simulink subsystem "ModeloSistemaNL"  (R2026a)
settings: Solver=VariableStepAuto
values from neighbouring files (symbols this model uses):
  alpha_Cu = 3.9e-3    (= 0.0039)    [coeficientes.m]
  b_eq = b_m + b_l/(r_m2l^2)    (= 2.19444444444e-05)    [coeficientes.m]
  C_ts = 0.818    [coeficientes.m]
  g = 9.80665    [coeficientes.m]
  J_eq = J_m + J_l/(r_m2l^2)    (= 4.58263888889e-05)    [coeficientes.m]
  k_l = 0.1    [coeficientes.m]
  L_d = 6.6e-3    (= 0.0066)    [coeficientes.m]
  L_ls = 0.8e-3    (= 0.0008)    [coeficientes.m]
  L_q = 5.8e-3    (= 0.0058)    [coeficientes.m]
  lambda = 0.016    [coeficientes.m]
  Pp = 3    [coeficientes.m]
  r_m2l = 120.0    (= 120)    [coeficientes.m]
  R_sREF = 1.02    [coeficientes.m]
  R_tsamb = 146.7    [coeficientes.m]
  T_amb = 20    [coeficientes.m]
  T_sREF = 20    [coeficientes.m]
libraries: eeTransforms x1
settings Model: Creator=barrios14101  LastModifiedBy=barrios14101

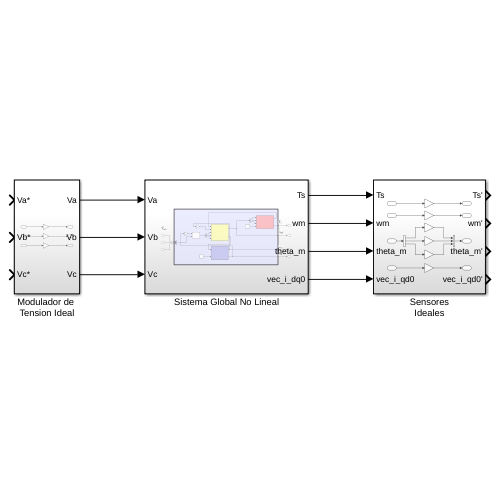
[thumbnail: Simulink's stored preview of the top-level diagram]
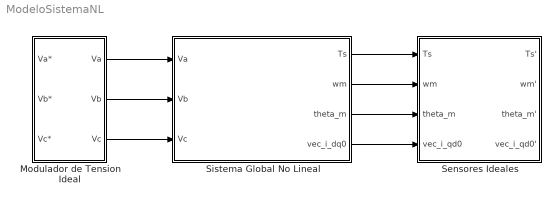
== system ModeloSistemaNL ==
  Modulador de Tension Ideal : Subsystem
  Sensores Ideales : Subsystem
  Sistema Global No Lineal : Subsystem
  wires:
  Modulador de Tension Ideal/1(Va) -> Sistema Global No Lineal/1(Va)
  Modulador de Tension Ideal/2(Vb) -> Sistema Global No Lineal/2(Vb)
  Modulador de Tension Ideal/3(Vc) -> Sistema Global No Lineal/3(Vc)
  Sistema Global No Lineal/1(Ts) -> Sensores Ideales/1(Ts)
  Sistema Global No Lineal/2(wm) -> Sensores Ideales/2(wm)
  Sistema Global No Lineal/3(theta_m) -> Sensores Ideales/3(theta_m)
  Sistema Global No Lineal/4(vec_i_dq0) -> Sensores Ideales/4(vec_i_qd0)

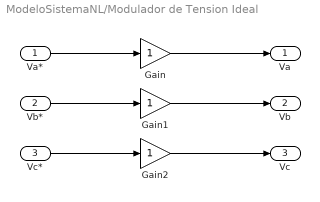
== system ModeloSistemaNL/Modulador de Tension Ideal ==
  Va* : Inport
  Vb* : Inport  Port=2
  Vc* : Inport  Port=3
  Gain : Gain
  Gain1 : Gain
  Gain2 : Gain
  Va : Outport
  Vb : Outport  Port=2
  Vc : Outport  Port=3
  wires:
  Va*/1 -> Gain/1
  Gain/1 -> Va/1
  Vb*/1 -> Gain1/1
  Gain1/1 -> Vb/1
  Vc*/1 -> Gain2/1
  Gain2/1 -> Vc/1

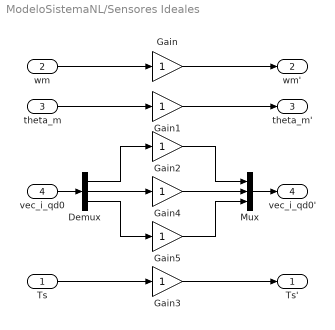
== system ModeloSistemaNL/Sensores Ideales ==
  Ts : Inport
  wm : Inport  Port=2
  theta_m : Inport  Port=3
  vec_i_qd0 : Inport  Port=4
  Demux : Demux  Outputs=3
  Gain{,1..5} (6 alike) : Gain
  Mux : Mux  Inputs=3
  Ts' : Outport
  wm' : Outport  Port=2
  theta_m' : Outport  Port=3
  vec_i_qd0' : Outport  Port=4
  wires:
  wm/1 -> Gain/1
  Gain/1 -> wm'/1
  theta_m/1 -> Gain1/1
  Gain1/1 -> theta_m'/1
  Ts/1 -> Gain3/1
  Gain3/1 -> Ts'/1
  vec_i_qd0/1 -> Demux/1
  Demux/2 -> Gain4/1
  Demux/1 -> Gain2/1
  Demux/3 -> Gain5/1
  Gain2/1 -> Mux/1
  Gain4/1 -> Mux/2
  Gain5/1 -> Mux/3
  Mux/1 -> vec_i_qd0'/1

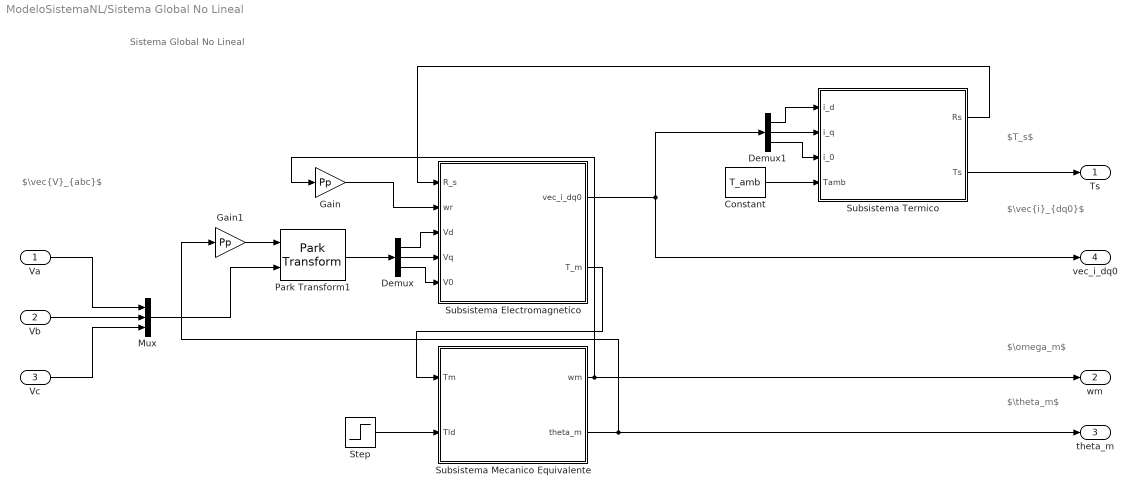
== system ModeloSistemaNL/Sistema Global No Lineal ==
  note: $\omega_m$
  note: $T_s$
  note: $\vec{i}_{dq0}$
  note: $\vec{V}_{abc}$
  note: Sistema Global No Lineal
  note: $\theta_m$
  Va : Inport
  Vb : Inport  Port=2
  Vc : Inport  Port=3
  Constant : Constant  Value=T_amb
  Demux : Demux  Outputs=3
  Demux1 : Demux  Outputs=3
  Gain : Gain  Gain=Pp
  Gain1 : Gain  Gain=Pp
  Mux : Mux  Inputs=3
  Park Transform1 : eeTransforms/Park Transform  AxisAlignment=D-axis  PowerInvariant=off
      settings: LibrarySourceBlock=|
      | ee_sl_lib/Mathematical
      | Transforms/Park Transform
  Step : Step  Time=0  FinalValue=15  SampleTime=0
  Subsistema Electromagnetico : Subsystem
  Subsistema Mecanico Equivalente : Subsystem
  Subsistema Termico : Subsystem
  Ts : Outport
  wm : Outport  Port=2
  theta_m : Outport  Port=3
  vec_i_dq0 : Outport  Port=4
  wires:
  Subsistema Termico/2(Ts) -> Ts/1
  Subsistema Electromagnetico/1(vec_i_dq0) -> vec_i_dq0/1, Demux1/1
  Subsistema Mecanico Equivalente/1(wm) -> wm/1, Gain/1
  Subsistema Mecanico Equivalente/2(theta_m) -> theta_m/1, Gain1/1
  Subsistema Electromagnetico/2(T_m) -> Subsistema Mecanico Equivalente/1(Tm)
  Demux1/2 -> Subsistema Termico/2(i_q)
  Subsistema Termico/1(Rs) -> Subsistema Electromagnetico/1(R_s)
  Park Transform1/1 -> Demux/1
  Gain1/1 -> Park Transform1/1
  Gain/1 -> Subsistema Electromagnetico/2(wr)
  Step/1 -> Subsistema Mecanico Equivalente/2(Tld)
  Va/1 -> Mux/1
  Mux/1 -> Park Transform1/2
  Demux1/1 -> Subsistema Termico/1(i_d)
  Vb/1 -> Mux/2
  Demux/3 -> Subsistema Electromagnetico/5(V0)
  Demux/2 -> Subsistema Electromagnetico/4(Vq)
  Demux/1 -> Subsistema Electromagnetico/3(Vd)
  Demux1/3 -> Subsistema Termico/3(i_0)
  Vc/1 -> Mux/3
  Constant/1 -> Subsistema Termico/4(Tamb)

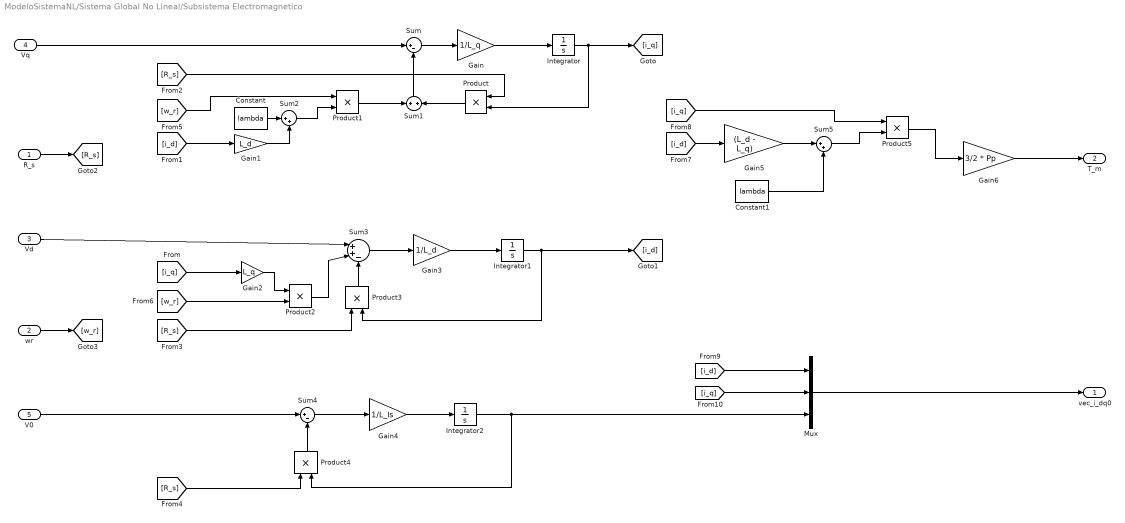
== system ModeloSistemaNL/Sistema Global No Lineal/Subsistema Electromagnetico ==
  R_s : Inport
  wr : Inport  Port=2
  Vd : Inport  Port=3
  Vq : Inport  Port=4
  V0 : Inport  Port=5
  Constant : Constant  Value=lambda
  Constant1 : Constant  Value=lambda
  Gain : Gain  Gain=1/L_q
  Gain1 : Gain  Gain=L_d
  Gain2 : Gain  Gain=L_q
  Gain3 : Gain  Gain=1/L_d
  Gain4 : Gain  Gain=1/L_ls
  Gain5 : Gain  Gain=(L_d - L_q)
  Gain6 : Gain  Gain=3/2 * Pp
  Integrator : Integrator
  Integrator1 : Integrator
  Integrator2 : Integrator
  Mux : Mux  Inputs=3
  Product{,1..5} (6 alike) : Product
  Sum : Sum  Inputs=|+-
  Sum1 : Sum
  Sum2 : Sum  Inputs=|++
  Sum3 : Sum  Inputs=|++-
  Sum4 : Sum  Inputs=|+-
  Sum5 : Sum  Inputs=|++
  vec_i_dq0 : Outport
  T_m : Outport  Port=2
  wires:
  Gain1/1 -> Sum2/2
  Product1/1 -> Sum1/1
  Sum2/1 -> Product1/2
  Constant/1 -> Sum2/1
  Product/1 -> Sum1/2
  Sum/1 -> Gain/1
  Sum1/1 -> Sum/2
  Vq/1 -> Sum/1
  Gain/1 -> Integrator/1
  Product3/1 -> Sum3/3
  Gain3/1 -> Integrator1/1
  Sum3/1 -> Gain3/1
  Product2/1 -> Sum3/2
  Gain2/1 -> Product2/1
  Vd/1 -> Sum3/1
  Product4/1 -> Sum4/2
  Integrator2/1 -> Product4/2, Mux/3
  Gain4/1 -> Integrator2/1
  Sum4/1 -> Gain4/1
  V0/1 -> Sum4/1
  Gain5/1 -> Sum5/1
  Sum5/1 -> Product5/2
  Integrator1/1 -> [i_d], Product3/2
  Constant1/1 -> Sum5/2
  Product5/1 -> Gain6/1
  Integrator/1 -> Product/2, [i_q]
  Gain6/1 -> T_m/1
  [i_q] -> Gain2/1
  [i_d] -> Gain1/1
  [R_s] -> Product/1
  R_s/1 -> [R_s]
  [R_s] -> Product3/1
  [R_s] -> Product4/1
  wr/1 -> [w_r]
  [w_r] -> Product1/1
  [w_r] -> Product2/2
  [i_d] -> Gain5/1
  [i_q] -> Product5/1
  [i_q] -> Mux/2
  [i_d] -> Mux/1
  Mux/1 -> vec_i_dq0/1

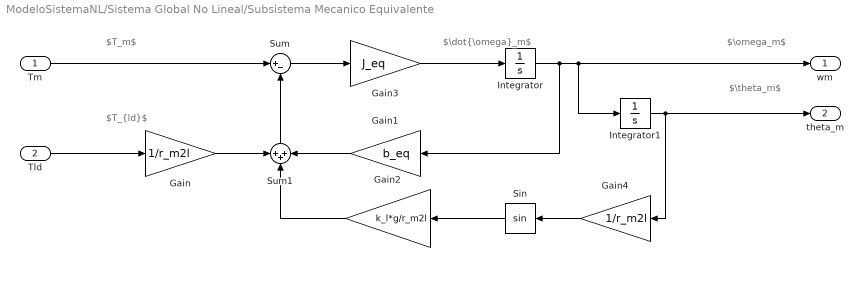
== system ModeloSistemaNL/Sistema Global No Lineal/Subsistema Mecanico Equivalente ==
  note: $T_m$
  note: $T_{ld}$
  note: $\dot{\omega}_m$
  note: $\omega_m$
  note: $\theta_m$
  Tm : Inport
  Tld : Inport  Port=2
  Gain : Gain  Gain=1/r_m2l
  Gain1 : Gain  Gain=b_eq
  Gain2 : Gain  Gain=k_l*g/r_m2l
  Gain3 : Gain  Gain=J_eq
  Gain4 : Gain  Gain=1/r_m2l
  Integrator : Integrator
  Integrator1 : Integrator
  Sin : Trigonometry
  Sum : Sum  Inputs=|+-
  Sum1 : Sum  Inputs=+++
  wm : Outport
  theta_m : Outport  Port=2
  wires:
  Integrator/1 -> Integrator1/1, wm/1, Gain1/1
  Integrator1/1 -> theta_m/1, Gain4/1
  Sum/1 -> Gain3/1
  Tm/1 -> Sum/1
  Sum1/1 -> Sum/2
  Gain2/1 -> Sum1/2
  Gain/1 -> Sum1/1
  Sin/1 -> Gain2/1
  Gain1/1 -> Sum1/3
  Gain3/1 -> Integrator/1
  Gain4/1 -> Sin/1
  Tld/1 -> Gain/1

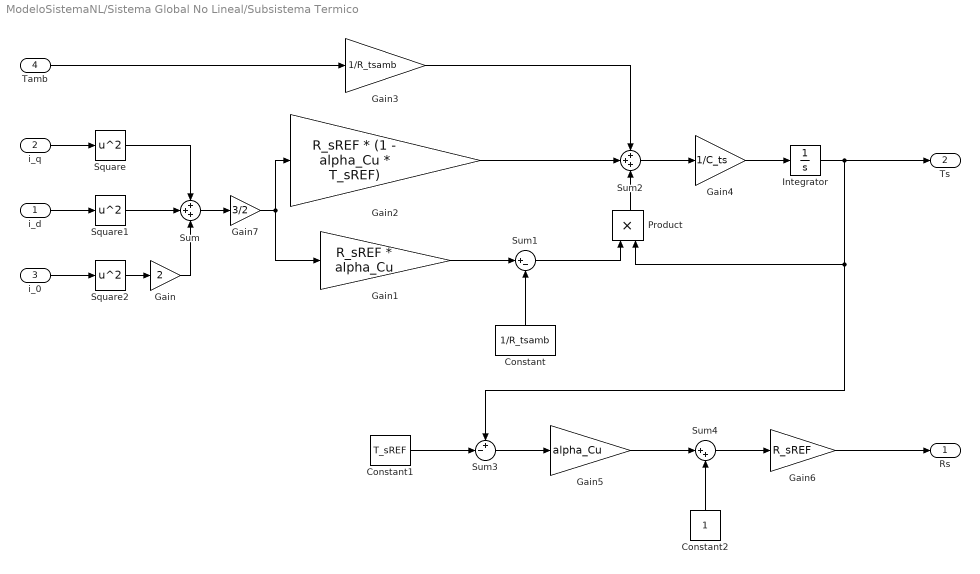
== system ModeloSistemaNL/Sistema Global No Lineal/Subsistema Termico ==
  i_d : Inport
  i_q : Inport  Port=2
  i_0 : Inport  Port=3
  Tamb : Inport  Port=4
  Constant : Constant  Value=1/R_tsamb
  Constant1 : Constant  Value=T_sREF
  Constant2 : Constant
  Gain : Gain  Gain=2
  Gain1 : Gain  Gain=R_sREF * alpha_Cu
  Gain2 : Gain  Gain="R_sREF * (1 -  alpha_Cu * T_sREF)"
  Gain3 : Gain  Gain=1/R_tsamb
  Gain4 : Gain  Gain=1/C_ts
  Gain5 : Gain  Gain=alpha_Cu
  Gain6 : Gain  Gain=R_sREF
  Gain7 : Gain  Gain=3/2
  Integrator : Integrator
  Product : Product
  Square : Math  Operator=square
  Square1 : Math  Operator=square
  Square2 : Math  Operator=square
  Sum : Sum  Inputs=+++
  Sum1 : Sum  Inputs=|+-
  Sum2 : Sum  Inputs=+++
  Sum3 : Sum  Inputs=+-|
  Sum4 : Sum  Inputs=|++
  Rs : Outport
  Ts : Outport  Port=2
  wires:
  Integrator/1 -> Sum3/1, Product/2, Ts/1
  Gain6/1 -> Rs/1
  Gain7/1 -> Gain2/1, Gain1/1
  Sum4/1 -> Gain6/1
  Constant1/1 -> Sum3/2
  Gain/1 -> Sum/3
  Gain5/1 -> Sum4/1
  Gain1/1 -> Sum1/1
  Constant/1 -> Sum1/2
  Sum3/1 -> Gain5/1
  Sum1/1 -> Product/1
  Tamb/1 -> Gain3/1
  Sum/1 -> Gain7/1
  Constant2/1 -> Sum4/2
  Square2/1 -> Gain/1
  Sum2/1 -> Gain4/1
  i_0/1 -> Square2/1
  i_d/1 -> Square1/1
  Square1/1 -> Sum/2
  Square/1 -> Sum/1
  Gain2/1 -> Sum2/2
  Gain4/1 -> Integrator/1
  Product/1 -> Sum2/3
  Gain3/1 -> Sum2/1
  i_q/1 -> Square/1
